simulink model "slToFlightgear"  (Simulink 7.9)
settings: Solver=ode4  StartTime=0.0  StopTime=-1  FixedStep=-1  RelTol=1e-3
InitFcn:
  | modelo2Initialization
undefined symbols (not defined in the file or in its folder): Earth, WGS84
libraries: simulink_extras x2, aerolibfltsims x2, aerolibtransform2 x1, aerolibanimutils x1
settings Model: Creator=claus  LastModifiedBy=claus
settings SolverCC: ShapePreserveControl=EnableAll
settings OptimizationCC: SimCompilerOptimization=On  AccelVerboseBuild=on
settings ModelReferenceCC: EnableParallelModelReferenceBuilds=on

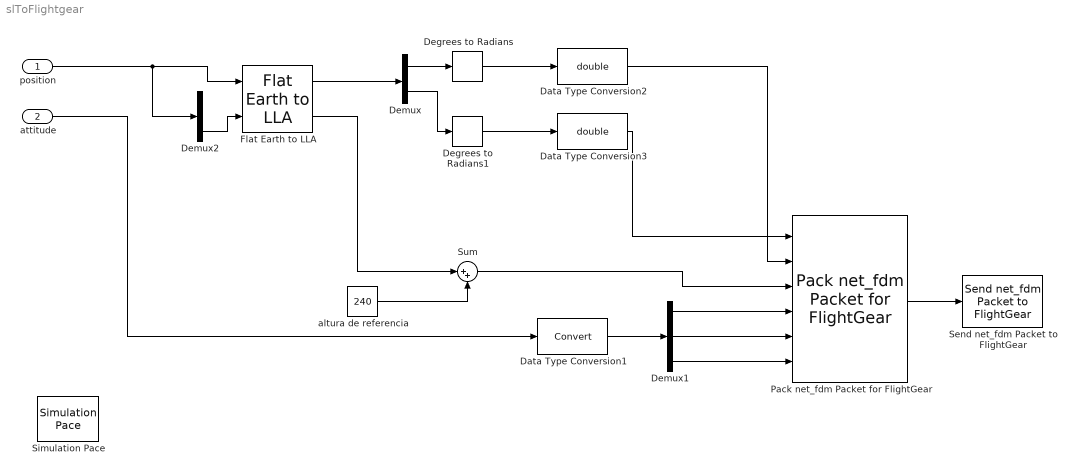
== system slToFlightgear ==
  position : Inport
  attitude : Inport  Port=2
  Data Type Conversion1 : DataTypeConversion
  Data Type Conversion2 : DataTypeConversion  OutDataTypeStr=double
  Data Type Conversion3 : DataTypeConversion  OutDataTypeStr=double
  Degrees to Radians : simulink_extras/Transformations/Degrees to Radians
  Degrees to Radians1 : simulink_extras/Transformations/Degrees to Radians
  Demux : Demux  Outputs=2
  Demux1 : Demux  Outputs=3
  Demux2 : Demux  Outputs=3
  Flat Earth to LLA : aerolibtransform2/Flat Earth to LLA  units=Metric (MKS)  ptype=Earth (WGS84)  F=1/298.257223563  R=6378137  LL0=[37.665543 -122.480847]  psi=0
  Pack net_fdm Packet for FlightGear : aerolibfltsims/Pack net_fdm Packet for FlightGear  FlightGearVersion=v2.0  ShowPositionAttitudeInputs=on  ShowVelocityAccelerationInputs=off  ShowControlSurfacePositionInputs=off  ShowEngineFuelInputs=off  ShowLandingGearInputs=off  ShowEnvironmentInputs=off  SampleTime=-1
  Send net_fdm Packet to FlightGear : aerolibfltsims/Send net_fdm Packet to FlightGear  DestinationIpAddress=127.0.0.1  DestinationPort=5502  LocalIpPort=-1  varLen=off  SampleTime=-1
  Simulation Pace : aerolibanimutils/Simulation Pace  SimulationPace=1  SleepMode=MATLAB Thread  OutputPaceError=off  SampleTime=0.1
      settings: AttributesFormatString=%<SimulationPace> sec/sec
  Sum : Sum  Inputs=|++
  altura de referencia : Constant  Value=240
  wires:
  position/1 -> Demux2/1, Flat Earth to LLA/1
  attitude/1 -> Data Type Conversion1/1
  Pack net_fdm Packet for FlightGear/1 -> Send net_fdm Packet to FlightGear/1
  Demux1/1 -> Pack net_fdm Packet for FlightGear/4
  Demux1/2 -> Pack net_fdm Packet for FlightGear/5
  Demux1/3 -> Pack net_fdm Packet for FlightGear/6
  Data Type Conversion1/1 -> Demux1/1
  Flat Earth to LLA/1 -> Demux/1
  Demux2/3 -> Flat Earth to LLA/2
  Degrees to Radians/1 -> Data Type Conversion2/1
  Degrees to Radians1/1 -> Data Type Conversion3/1
  Demux/1 -> Degrees to Radians/1
  Demux/2 -> Degrees to Radians1/1
  Data Type Conversion3/1 -> Pack net_fdm Packet for FlightGear/1
  Data Type Conversion2/1 -> Pack net_fdm Packet for FlightGear/2
  Flat Earth to LLA/2 -> Sum/1
  altura de referencia/1 -> Sum/2
  Sum/1 -> Pack net_fdm Packet for FlightGear/3
